simulink model "demo1"  (R2025a)
settings: Solver=VariableStepAuto  StartTime=0.0  StopTime=10.0  RelTol=1e-3
libraries: StdLib x5
settings Model: Creator=peter  LastModifiedBy=peter

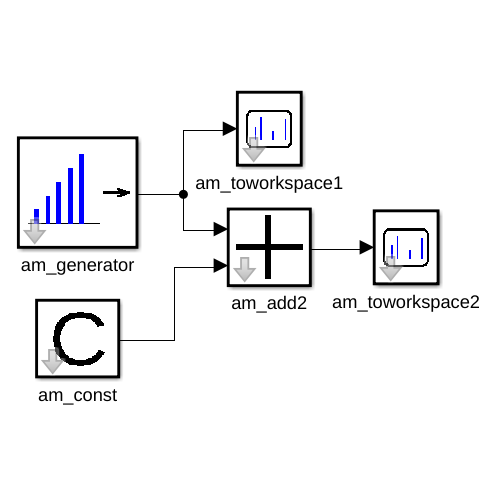
[thumbnail: Simulink's stored preview of the top-level diagram]
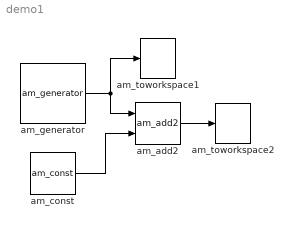
== system demo1 ==
  am_add2 : StdLib/am_add2  tau=[0,1]  debug=0
  am_const : StdLib/am_const  value=3  sendTime=[0,1]  debug=0
      settings: SourceProductName=Sources
  am_generator : StdLib/am_generator  tG=1  n0=1  nG=inf  tD=[0,2]  debug=0
  am_toworkspace1 : StdLib/am_toworkspace  varname="\"input\""  t0=0  format="\"vector\""  tau=[0,5]  debug=0
  am_toworkspace2 : StdLib/am_toworkspace  varname="\"result\""  t0=0  format="\"vector\""  tau=[0,5]  debug=0
  wires:
  am_const/1 -> am_add2/2
  am_generator/1 -> am_add2/1, am_toworkspace1/1
  am_add2/1 -> am_toworkspace2/1
